simulink model "control_lab3_simulink"  (R2023b)
settings: Solver=VariableStepAuto  StartTime=0.0  StopTime=10.0  RelTol=1e-3
values from neighbouring files (symbols this model uses):
  b = a*2    (= 2)    [airLabTest.m]    (also in control_lab2_1.m = 0.1; control_lab2_2.m = 0.1; control_lab2_assign.m = 0.1; control_lab3_simulink.m = 0.1)
  g = 1.4    [airDyn2_HW4.m]    (also in control_lab2_1.m = 9.8; control_lab2_2.m = 9.8; control_lab2_assign.m = 9.8; control_lab3_simulink.m = 9.8)
  I = 0.006    [control_lab2_1.m]    (also in control_lab2_2.m; control_lab2_assign.m; control_lab3_simulink.m)
  l = linspace(0,2,nl)    [HW3_3D_Foil_Generator.m]    (also in control_lab3_simulink.m = 0.3)
  m = (1/10)*str2double(digit(2))    [HW3_3D_Foil_Generator.m]    (also in airDyn2_HW4.m = 1; control_lab1.m = 2; control_lab1_assign.m = 2; control_lab2_1.m = 0.2)
  M = 0.5    [control_lab2_1.m]    (also in control_lab2_2.m; control_lab2_assign.m; control_lab3_simulink.m)
settings Model: Creator=henry  LastModifiedBy=henry

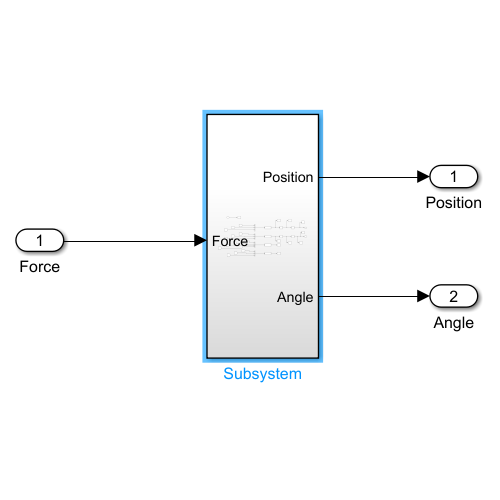
[thumbnail: Simulink's stored preview of the top-level diagram]
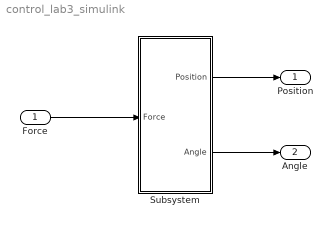
== system control_lab3_simulink ==
  Force : Inport
  Subsystem : Subsystem
  Position : Outport
  Angle : Outport  Port=2
  wires:
  Force/1 -> Subsystem/1(Force)
  Subsystem/1(Position) -> Position/1
  Subsystem/2(Angle) -> Angle/1

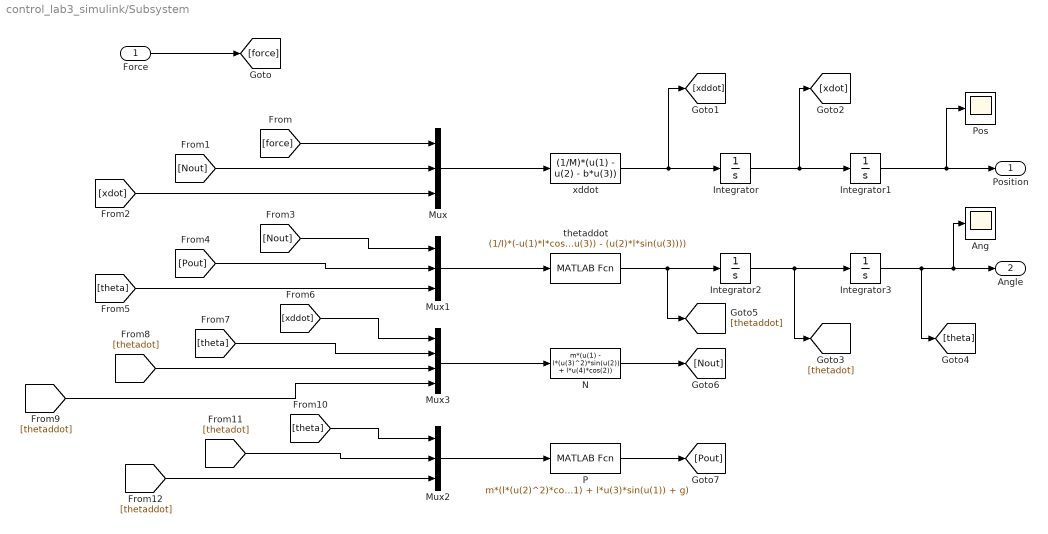
== system control_lab3_simulink/Subsystem ==
  Force : Inport
  Ang : Scope
  Integrator{,1..3} (4 alike) : Integrator
  Mux : Mux  Inputs=3
  Mux1 : Mux  Inputs=3
  Mux2 : Mux  Inputs=3
  Mux3 : Mux
  N : MATLABFcn  MATLABFcn=m*(u(1) - l*(u(3)^2)*sin(u(2)) + l*u(4)*cos(2))
  P : MATLABFcn  MATLABFcn=m*(l*(u(2)^2)*cos(1) + l*u(3)*sin(u(1)) + g)
  Pos : Scope
  thetaddot : MATLABFcn  MATLABFcn=(1/I)*(-u(1)*l*cos(u(3)) - (u(2)*l*sin(u(3))))
  xddot : MATLABFcn  MATLABFcn=(1/M)*(u(1) - u(2) - b*u(3))
  Position : Outport
  Angle : Outport  Port=2
  wires:
  thetaddot/1 -> [thetaddot], Integrator2/1
  N/1 -> [Nout]
  Integrator1/1 -> Pos/1, Position/1
  xddot/1 -> [xddot], Integrator/1
  Integrator/1 -> [xdot], Integrator1/1
  Mux2/1 -> P/1
  [theta] -> Mux3/2
  Mux3/1 -> N/1
  [Pout] -> Mux1/2
  [xddot] -> Mux3/1
  [force] -> Mux/1
  [thetadot] -> Mux3/3
  [theta] -> Mux2/1
  Integrator2/1 -> [thetadot], Integrator3/1
  Integrator3/1 -> Ang/1, Angle/1, [theta]
  [thetadot] -> Mux2/2
  [thetaddot] -> Mux2/3
  [xdot] -> Mux/3
  [theta] -> Mux1/3
  [Nout] -> Mux1/1
  [Nout] -> Mux/2
  Mux/1 -> xddot/1
  [thetaddot] -> Mux3/4
  Force/1 -> [force]
  Mux1/1 -> thetaddot/1
  P/1 -> [Pout]
